simulink model "GuidePT1"  (R2016a)
settings: Solver=VariableStepAuto  StartTime=0.0  StopTime=10.0  RelTol=1e-3
settings Model: Creator=Michaél  LastModifiedBy=Michaél

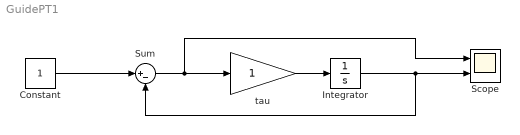
== system GuidePT1 ==
  Constant : Constant
  Integrator : Integrator
  Scope : Scope  NumInputPorts=2
  Sum : Sum  Inputs=|+-
  tau : Gain
  wires:
  Constant/1 -> Sum/1
  Sum/1 -> Scope/1, tau/1
  tau/1 -> Integrator/1
  Integrator/1 -> Sum/2, Scope/2
